simulink model "fourinputslq_and_yaw_rate_control_sim"  (R2015a)
settings: Solver=ode3  SolverMode=SingleTasking  StartTime=0.0  StopTime=5  FixedStep=ts  RelTol=1e-3
values from neighbouring files (symbols this model uses):
  A = eval(As)    [fourinputslq_and_yaw_rate_control.m]    (also in matlab.mat = [0 0 0 1 0 0 0 0 0 0 1 0 ... (36 elements, 6x6)])
  B = eval(Bs)    [fourinputslq_and_yaw_rate_control.m]    (also in matlab.mat = [-77.4114285714 -77.4114285714 0.00460829493088 0 0 0 -77.41)
  Cc = [0 0 1 0 0; 0 0 0 1 0; 0 0 0 0 1 ]    [fourinputslq_and_yaw_rate_control.m]    (also in matlab.mat = [0 0 0 0 0 0 1 0 0 0 1 0 ... (15 elements, 3x5)])
  Cs = [1 0 0 0 0 0; 0 1 0 0 0 0; 0 0 1 0 0 0;  0 0 0 1 0 0;0 0 0 0 1 0]    [fourinputslq_and_yaw_rate_control.m]    (also in matlab.mat = [1 0 0 0 0 0 1 0 0 0 0 0 ... (30 elements, 5x6)])
  Kd = [-0.106033848102 -0.106033848102 0.106033848102 0.106033848102 -0.106033848102 0.106033848102 0.106033848102 -0.106033848102 414.166107051 -414.166107051 414.166107051 -414.166107051 ... (32 elements, 4x8)]    [matlab.mat]
  ts = 1/250    (= 0.004)    [fourinputslq_and_yaw_rate_control.m]    (also in matlab.mat)
undefined symbols (not defined in the file or in its folder): K
settings Model: Creator=Jaby  LastModifiedBy=Jaby
settings OptimizationCC: BlockReduction=off  BooleanDataType=off
settings DebuggingCC: SaveWithParameterizedLinksMsg=none  UnderspecifiedInitializationDetection=Classic  MergeDetectMultiDrivingBlocksExec=none  SignalResolutionControl=TryResolveAllWithWarning
settings HardwareCC: TargetUnknown=on

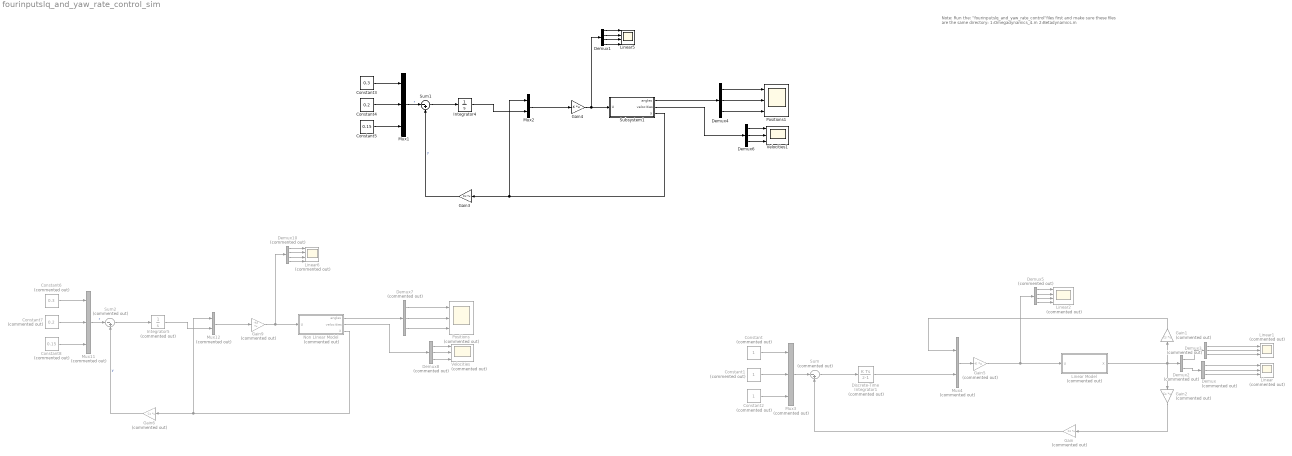
== system fourinputslq_and_yaw_rate_control_sim ==
  note: Note:
      | Run the: "fourinputslq_and_yaw_rate_control"files first and make sure these files are the same directory:
      | 1:Omegadynamics_4.m
      | 2:Betadynamics.m
  Constant : Constant  Commented=on  VectorParams1D=off
  Constant1 : Constant  Commented=on
  Constant2 : Constant  Commented=on  VectorParams1D=off
  Constant3 : Constant  Value=0.3  VectorParams1D=off
  Constant4 : Constant  Value=0.2  VectorParams1D=off
  Constant5 : Constant  Value=0.15  VectorParams1D=off
  Constant6 : Constant  Commented=on  Value=0.3  VectorParams1D=off
  Constant7 : Constant  Commented=on  Value=0.2  VectorParams1D=off
  Constant8 : Constant  Commented=on  Value=0.15  VectorParams1D=off
  Demux{,3,7..8} (4 alike) : Demux  Commented=on  Outputs=3
  Demux1 : Demux
  Demux10 : Demux  Commented=on
  Demux2 : Demux  Commented=on  Outputs=2
  Demux4 : Demux  Outputs=3
  Demux5 : Demux  Commented=on
  Demux6 : Demux  Outputs=3
  Discrete-Time Integrator1 : DiscreteIntegrator  Commented=on  InitialConditionSetting=State (most efficient)  SampleTime=ts
  Gain : Gain  Commented=on  Gain=Cc  Multiplication=Matrix(K*u)
  Gain1 : Gain  Commented=on  Gain=Cs  Multiplication=Matrix(K*u)
  Gain2 : Gain  Commented=on  Gain=Cs  Multiplication=Matrix(K*u)
  Gain3 : Gain  Gain=Cc  Multiplication=Matrix(K*u)
  Gain4 : Gain  Gain=-K  Multiplication=Matrix(K*u)
  Gain5 : Gain  Commented=on  Gain=-K  Multiplication=Matrix(K*u)
  Gain6 : Gain  Commented=on  Gain=Cc  Multiplication=Matrix(K*u)
  Gain9 : Gain  Commented=on  Gain=-Kd  Multiplication=Matrix(K*u)
  Integrator4 : Integrator  InitialCondition=[0 0 0]'
  Integrator5 : Integrator  Commented=on  InitialCondition=[0 0 0]'
  Linear : Scope  Commented=on  NumInputPorts=3
      settings: TimeRange=8.736052223432505  YMin=2.975e-07~-1~-1  YMax=3.325e-07~1~1
  "Linear Model " : Subsystem  Commented=on
  Linear1 : Scope  Commented=on  NumInputPorts=3
      settings: TimeRange=10  YMin=-0.5~-0.5~0  YMax=3.5~3.5~1.2  SaveName=ScopeData2
  Linear2 : Scope  Commented=on  NumInputPorts=4
      settings: TimeRange=20  YMin=-100000~-100000~-50000~-50000  YMax=50000~50000~100000~100000  SaveName=ScopeData4
  Linear5 : Scope  NumInputPorts=4
      settings: TimeRange=20  YMin=0.00274~-3.07e-14~8.3e-31~-5  YMax=0.00278~-3.025e-14~8.43e-31~5  SaveName=ScopeData3
  Linear6 : Scope  Commented=on  NumInputPorts=4
      settings: TimeRange=20  YMin=0.00274~-3.07e-14~8.3e-31~-5  YMax=0.00278~-3.025e-14~8.43e-31~5  SaveName=ScopeData10
  Mux1 : Mux  Inputs=3
  Mux11 : Mux  Commented=on  Inputs=3
  Mux12 : Mux  Commented=on  Inputs=2
  Mux2 : Mux  Inputs=2
  Mux3 : Mux  Commented=on  Inputs=3
  Mux4 : Mux  Commented=on  Inputs=2
  "Non LInear Model " : Subsystem  Commented=on
  Positions : Scope  Commented=on  NumInputPorts=3
      settings: TimeRange=30  YMin=-5e-19~-2e-19~0  YMax=1e-18~8.000000000000001e-19~8  SaveName=ScopeData7
  Positions1 : Scope  NumInputPorts=3
      settings: TimeRange=30  YMin=-5e-19~-2e-19~0  YMax=1e-18~8.000000000000001e-19~8  SaveName=ScopeData5
  Subsystem1 : Subsystem
  Sum : Sum  Commented=on  Inputs=|-+
  Sum1 : Sum  Inputs=|-+
  Sum2 : Sum  Commented=on  Inputs=|-+
  Velocities : Scope  Commented=on  NumInputPorts=3
      settings: YMin=-5~-5~-5  YMax=5~5~5  SaveName=ScopeData8
  Velocities1 : Scope  NumInputPorts=3
      settings: YMin=-5~-5~-5  YMax=5~5~5  SaveName=ScopeData9
  wires:
  Demux/1 -> Linear/1
  Demux/2 -> Linear/2
  Demux/3 -> Linear/3
  Gain/1 -> Sum/2
  Demux2/2 -> Demux/1
  Constant1/1 -> Mux3/2
  Constant/1 -> Mux3/1
  Demux3/1 -> Linear1/1
  Demux3/2 -> Linear1/2
  Demux3/3 -> Linear1/3
  Constant2/1 -> Mux3/3
  "Linear Model "/1(X) -> Gain2/1, Demux2/1, Gain1/1
  Mux3/1 -> Sum/1
  Gain2/1 -> Gain/1
  Demux2/1 -> Demux3/1
  Sum/1 -> Discrete-Time Integrator1/1
  Gain1/1 -> Mux4/1
  Mux4/1 -> Gain5/1
  Discrete-Time Integrator1/1 -> Mux4/2
  Demux5/1 -> Linear2/1
  Demux5/2 -> Linear2/2
  Demux5/3 -> Linear2/3
  Demux5/4 -> Linear2/4
  Gain5/1 -> "Linear Model "/1(U), Demux5/1
  Demux7/2 -> Positions/2
  Demux7/3 -> Positions/3
  Demux7/1 -> Positions/1
  Gain6/1 -> Sum2/2  "y"
  Demux8/2 -> Velocities/2
  Demux8/3 -> Velocities/3
  Demux8/1 -> Velocities/1
  Constant7/1 -> Mux11/2
  Constant6/1 -> Mux11/1
  Constant8/1 -> Mux11/3
  Mux11/1 -> Sum2/1  "r"
  Sum2/1 -> Integrator5/1
  Integrator5/1 -> Mux12/2
  Mux12/1 -> Gain9/1
  Demux10/1 -> Linear6/1
  Demux10/2 -> Linear6/2
  Demux10/3 -> Linear6/3
  Demux10/4 -> Linear6/4
  "Non LInear Model "/3(X) -> Gain6/1, Mux12/1
  "Non LInear Model "/1(angles) -> Demux7/1
  "Non LInear Model "/2(velocities) -> Demux8/1
  Gain9/1 -> Demux10/1, "Non LInear Model "/1(U)
  Demux4/2 -> Positions1/2
  Demux4/3 -> Positions1/3
  Demux4/1 -> Positions1/1
  Gain3/1 -> Sum1/2  "y"
  Demux6/2 -> Velocities1/2
  Demux6/3 -> Velocities1/3
  Demux6/1 -> Velocities1/1
  Constant4/1 -> Mux1/2
  Constant3/1 -> Mux1/1
  Constant5/1 -> Mux1/3
  Mux1/1 -> Sum1/1  "r"
  Demux1/1 -> Linear5/1
  Demux1/2 -> Linear5/2
  Demux1/3 -> Linear5/3
  Demux1/4 -> Linear5/4
  Subsystem1/3(X) -> Mux2/1, Gain3/1
  Subsystem1/1(angles) -> Demux4/1
  Subsystem1/2(velocities) -> Demux6/1
  Gain4/1 -> Subsystem1/1(U), Demux1/1
  Mux2/1 -> Gain4/1
  Sum1/1 -> Integrator4/1
  Integrator4/1 -> Mux2/2

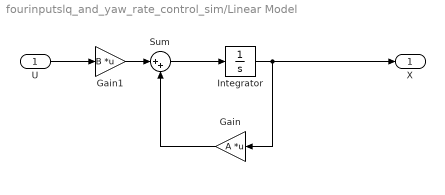
== system fourinputslq_and_yaw_rate_control_sim/Linear Model  ==
  U : Inport
  Gain : Gain  Gain=A  Multiplication=Matrix(K*u)
  Gain1 : Gain  Gain=B  Multiplication=Matrix(K*u)
  Integrator : Integrator
  Sum : Sum  Inputs=|++
  X : Outport
  wires:
  Integrator/1 -> X/1, Gain/1
  U/1 -> Gain1/1
  Gain1/1 -> Sum/1
  Sum/1 -> Integrator/1
  Gain/1 -> Sum/2

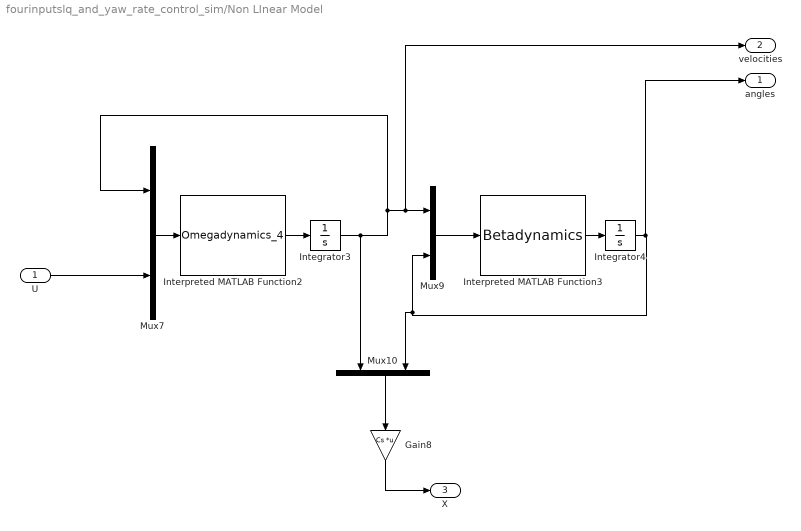
== system fourinputslq_and_yaw_rate_control_sim/Non LInear Model  ==
  U : Inport
  Gain8 : Gain  Gain=Cs  Multiplication=Matrix(K*u)
  Integrator3 : Integrator  InitialCondition=[0 0 0]'
  Integrator4 : Integrator  InitialCondition=[0 0 0]'
  Interpreted MATLAB Function2 : MATLABFcn  MATLABFcn=Omegadynamics_4  Output1D=off
  Interpreted MATLAB Function3 : MATLABFcn  MATLABFcn=Betadynamics  Output1D=off
  Mux10 : Mux  Inputs=2
  Mux7 : Mux  Inputs=2
  Mux9 : Mux  Inputs=2
  angles : Outport
  velocities : Outport  Port=2
  X : Outport  Port=3
  wires:
  Integrator3/1 -> Mux7/1, velocities/1, Mux9/1, Mux10/1
  Mux7/1 -> Interpreted MATLAB Function2/1
  Interpreted MATLAB Function2/1 -> Integrator3/1
  Interpreted MATLAB Function3/1 -> Integrator4/1
  Mux10/1 -> Gain8/1
  Mux9/1 -> Interpreted MATLAB Function3/1
  Integrator4/1 -> angles/1, Mux9/2, Mux10/2
  U/1 -> Mux7/2
  Gain8/1 -> X/1

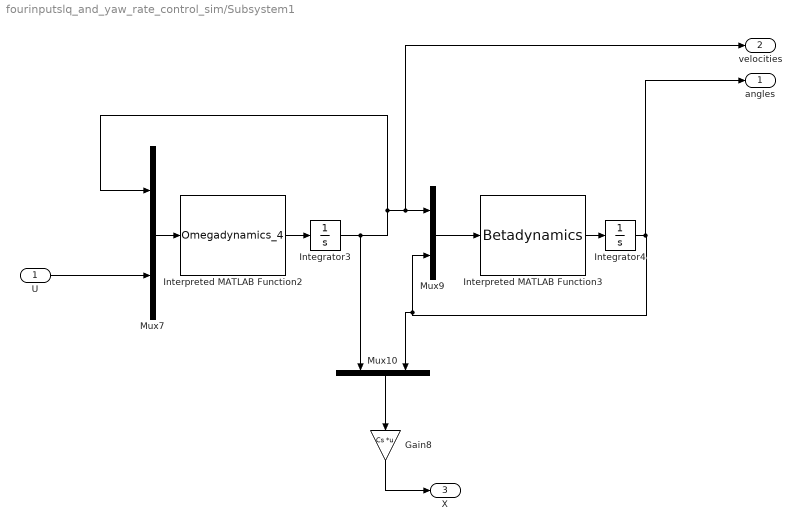
== system fourinputslq_and_yaw_rate_control_sim/Subsystem1 ==
  U : Inport
  Gain8 : Gain  Gain=Cs  Multiplication=Matrix(K*u)
  Integrator3 : Integrator  InitialCondition=[0 0 0]'
  Integrator4 : Integrator  InitialCondition=[0 0 0]'
  Interpreted MATLAB Function2 : MATLABFcn  MATLABFcn=Omegadynamics_4  Output1D=off
  Interpreted MATLAB Function3 : MATLABFcn  MATLABFcn=Betadynamics  Output1D=off
  Mux10 : Mux  Inputs=2
  Mux7 : Mux  Inputs=2
  Mux9 : Mux  Inputs=2
  angles : Outport
  velocities : Outport  Port=2
  X : Outport  Port=3
  wires:
  Gain8/1 -> X/1
  U/1 -> Mux7/2
  Integrator4/1 -> Mux10/2, Mux9/2, angles/1
  Mux9/1 -> Interpreted MATLAB Function3/1
  Mux10/1 -> Gain8/1
  Interpreted MATLAB Function3/1 -> Integrator4/1
  Interpreted MATLAB Function2/1 -> Integrator3/1
  Mux7/1 -> Interpreted MATLAB Function2/1
  Integrator3/1 -> Mux10/1, Mux9/1, velocities/1, Mux7/1
